simulink model "assignment_4"  (R2020b)
settings: Solver=VariableStepAuto  StartTime=0  StopTime=10  FixedStep=1  MaxStep=1  RelTol=1e-3
settings Model: Creator=Sudhanshu  LastModifiedBy=Sudhanshu

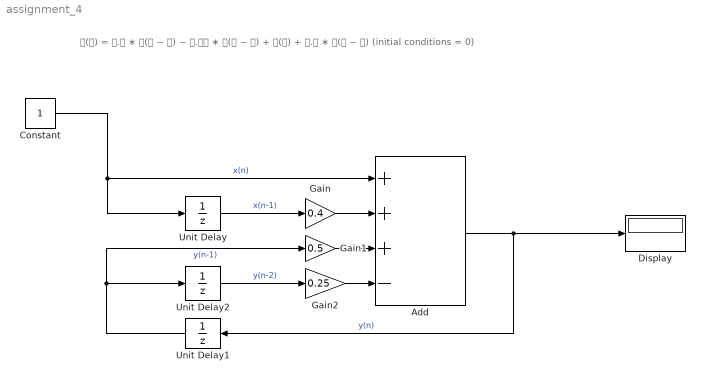
== system assignment_4 ==
  note: 𝐲(𝐧) = 𝟎.𝟓 ∗ 𝐲(𝐧 − 𝟏) − 𝟎.𝟐𝟓 ∗ 𝐲(𝐧 − 𝟐) + 𝐱(𝐧) + 𝟎.𝟒 ∗ 𝐱(𝐧 − 𝟏)
      |
      | (initial conditions = 0)
  Add : Sum  Inputs=+++-
  Constant : Constant
  Display : Display
  Gain : Gain  Gain=0.4
  Gain1 : Gain  Gain=0.5
  Gain2 : Gain  Gain=0.25
  Unit Delay : UnitDelay  SampleTime=-1  HasFrameUpgradeWarning=on
  Unit Delay1 : UnitDelay  SampleTime=-1  HasFrameUpgradeWarning=on
  Unit Delay2 : UnitDelay  SampleTime=-1  HasFrameUpgradeWarning=on
  wires:
  Constant/1 -> Unit Delay/1, Add/1  "x(n)"
  Unit Delay/1 -> Gain/1  "x(n-1)"
  Add/1 -> Unit Delay1/1, Display/1  "y(n)"
  Gain/1 -> Add/2
  Unit Delay1/1 -> Gain1/1, Unit Delay2/1  "y(n-1)"
  Gain1/1 -> Add/3
  Unit Delay2/1 -> Gain2/1  "y(n-2)"
  Gain2/1 -> Add/4
